simulink model "Linear_observer_MPC_controller"  (R2022a)
settings: Solver=VariableStepAuto  StartTime=0.0  StopTime=10000  RelTol=1e-3
values from neighbouring files (symbols this model uses):
  A = [0 0 0 ... (first row only)    [Lithium_ion_oneCell_Modeling_continuous_Linear.m]    (also in Lithium_ion_oneCell_Modeling_continuous_new.m)
  A_aug = [A_d zeros(3,1);C_d*A_d 1]    [Lithium_ion_oneCell_Modeling_continuous_Linear.m]
  B = [-eta/C_max ... (first row only)    [Lithium_ion_oneCell_Modeling_continuous_Linear.m]    (also in Lithium_ion_oneCell_Modeling_continuous_new.m)
  B_aug = [B_d;C_d*B_d+D_d]    [Lithium_ion_oneCell_Modeling_continuous_Linear.m]
  C = [0.5672 -1 -1]    [Lithium_ion_oneCell_Modeling_continuous_Linear.m]    (also in Lithium_ion_oneCell_Modeling_continuous_new.m = [0 -1 -1])
  C_aug = [zeros(1,3) 1]    [Lithium_ion_oneCell_Modeling_continuous_Linear.m]
  D_aug = D_d    [Lithium_ion_oneCell_Modeling_continuous_Linear.m]
  K_mpc = [1 zeros(1,N_c-1)]*inv(H)*Phi_F    [Lithium_ion_oneCell_Modeling_continuous_Linear.m]
  K_r = [1 zeros(1,N_c-1)]*inv(H)*Phi_R    [Lithium_ion_oneCell_Modeling_continuous_Linear.m]
  L = acker(A_d',C_d',[0.001,0.001,0.001])'    [Lithium_ion_oneCell_Modeling_continuous_Linear.m]
  L_aug = acker(A_aug', C_aug',[0.001,0.001,0.001,0.001])'    [Lithium_ion_oneCell_Modeling_continuous_Linear.m]
  X0 = [0.6; 0; 0]    [Lithium_ion_oneCell_Modeling_continuous_Linear.m]    (also in Lithium_ion_oneCell_Modeling_continuous_new.m = [0.6;0;0])
  x0 = [0;0;0;0]    [Lithium_ion_oneCell_Modeling_continuous_Linear.m]
libraries: simulink x1
settings Model: Creator=Asus  LastModifiedBy=Asus

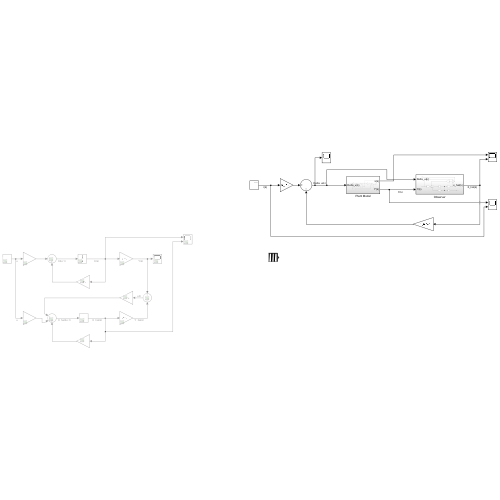
[thumbnail: Simulink's stored preview of the top-level diagram]
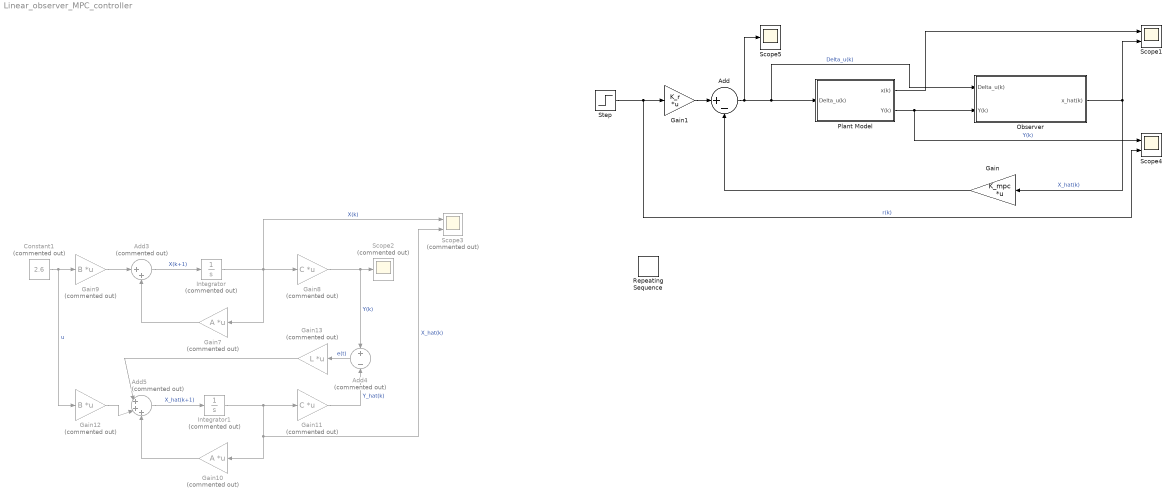
== system Linear_observer_MPC_controller ==
  Add : Sum  Inputs=|+-
  Add3 : Sum  Commented=on  Inputs=|++
  Add4 : Sum  Commented=on  Inputs=+-
  Add5 : Sum  Commented=on  Inputs=|+++
  Constant1 : Constant  Commented=on  Value=2.6
  Gain : Gain  Gain=K_mpc  Multiplication=Matrix(K*u)
  Gain1 : Gain  Gain=K_r  Multiplication=Matrix(K*u)
  Gain10 : Gain  Commented=on  Gain=A  Multiplication=Matrix(K*u)
  Gain11 : Gain  Commented=on  Gain=C  Multiplication=Matrix(K*u)
  Gain12 : Gain  Commented=on  Gain=B  Multiplication=Matrix(K*u)
  Gain13 : Gain  Commented=on  Gain=L  Multiplication=Matrix(K*u)
  Gain7 : Gain  Commented=on  Gain=A  Multiplication=Matrix(K*u)
  Gain8 : Gain  Commented=on  Gain=C  Multiplication=Matrix(K*u)
  Gain9 : Gain  Commented=on  Gain=B  Multiplication=Matrix(K*u)
  Integrator : Integrator  Commented=on  InitialCondition=X0
  Integrator1 : Integrator  Commented=on
  Observer : Subsystem
  Plant Model : Subsystem
  Repeating Sequence : simulink/Sources/Repeating Sequence  rep_seq_t=[0 2 4 6 8 10]  rep_seq_y=[0 2 2 2 2 2]
  Scope1 : Scope  NumInputPorts=2
  Scope2 : Scope  Commented=on
  Scope3 : Scope  Commented=on  NumInputPorts=2
  Scope4 : Scope  NumInputPorts=2
  Scope5 : Scope
  Step : Step  Time=10000  After=5  SampleTime=0
  wires:
  Add/1 -> Scope5/1, Observer/1(Delta_u(k)), Plant Model/1(Delta_u(k))  "Delta_u(k)"
  Gain13/1 -> Add5/1
  Gain12/1 -> Add5/2
  Add5/1 -> Integrator1/1  "X_hat(k+1)"
  Add4/1 -> Gain13/1  "e(t)"
  Constant1/1 -> Gain12/1, Gain9/1  "u"
  Integrator1/1 -> Gain10/1, Scope3/2, Gain11/1  "X_hat(k)"
  Gain10/1 -> Add5/3
  Gain9/1 -> Add3/1
  Gain7/1 -> Add3/2
  Integrator/1 -> Scope3/1, Gain7/1, Gain8/1  "X(k)"
  Gain8/1 -> Add4/1, Scope2/1  "Y(k)"
  Gain11/1 -> Add4/2  "Y_hat(k)"
  Add3/1 -> Integrator/1  "X(k+1)"
  Plant Model/1(x(k)) -> Scope1/1
  Plant Model/2(Y(k)) -> Scope4/1, Observer/2(Y(k))  "Y(k)"
  Observer/1(x_hat(k)) -> Gain/1, Scope1/2  "X_hat(k)"
  Step/1 -> Gain1/1, Scope4/2  "r(k)"
  Gain/1 -> Add/2
  Gain1/1 -> Add/1

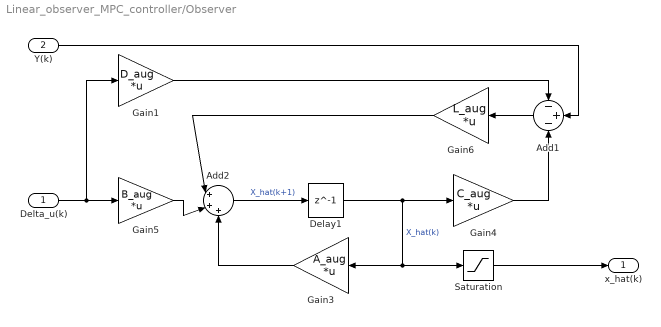
== system Linear_observer_MPC_controller/Observer ==
  Delta_u(k) : Inport
  Y(k) : Inport  Port=2
  Add1 : Sum  Inputs=-+-
  Add2 : Sum  Inputs=|+++
  Delay1 : Delay  DelayLength=1  InitialCondition=0
  Gain1 : Gain  Gain=D_aug  Multiplication=Matrix(K*u)
  Gain3 : Gain  Gain=A_aug  Multiplication=Matrix(K*u)
  Gain4 : Gain  Gain=C_aug  Multiplication=Matrix(K*u)
  Gain5 : Gain  Gain=B_aug  Multiplication=Matrix(K*u)
  Gain6 : Gain  Gain=L_aug  Multiplication=Matrix(K*u)
  Saturation : Saturate  UpperLimit=[1;4.2;4.2;10]  LowerLimit=0
  x_hat(k) : Outport
  wires:
  Delay1/1 -> Saturation/1, Gain3/1, Gain4/1  "X_hat(k)"
  Add1/1 -> Gain6/1
  Gain5/1 -> Add2/2
  Gain3/1 -> Add2/3
  Delta_u(k)/1 -> Gain1/1, Gain5/1
  Gain6/1 -> Add2/1
  Add2/1 -> Delay1/1  "X_hat(k+1)"
  Y(k)/1 -> Add1/2
  Gain4/1 -> Add1/3
  Gain1/1 -> Add1/1
  Saturation/1 -> x_hat(k)/1

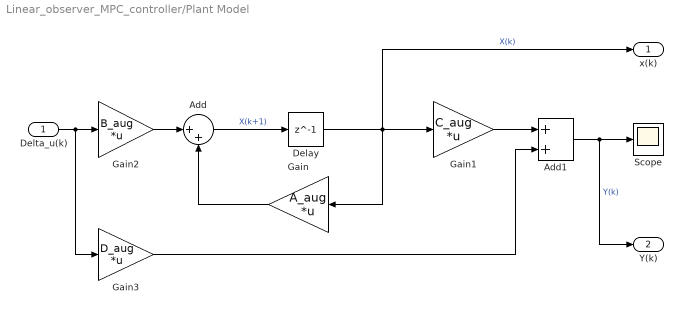
== system Linear_observer_MPC_controller/Plant Model ==
  Delta_u(k) : Inport
  Add : Sum  Inputs=|++
  Add1 : Sum
  Delay : Delay  DelayLength=1  InitialCondition=x0
  Gain : Gain  Gain=A_aug  Multiplication=Matrix(K*u)
  Gain1 : Gain  Gain=C_aug  Multiplication=Matrix(K*u)
  Gain2 : Gain  Gain=B_aug  Multiplication=Matrix(K*u)
  Gain3 : Gain  Gain=D_aug  Multiplication=Matrix(K*u)
  Scope : Scope
  x(k) : Outport
  Y(k) : Outport  Port=2
  wires:
  Delay/1 -> Gain/1, Gain1/1, x(k)/1  "X(k)"
  Gain/1 -> Add/2
  Delta_u(k)/1 -> Gain2/1, Gain3/1
  Add/1 -> Delay/1  "X(k+1)"
  Gain2/1 -> Add/1
  Gain1/1 -> Add1/1
  Add1/1 -> Y(k)/1, Scope/1  "Y(k)"
  Gain3/1 -> Add1/2
